simulink model "unit2"  (R2020a)
settings: Solver=VariableStepAuto  StartTime=0.0  StopTime=10.0  RelTol=1e-3
settings Model: Creator=fsepcke  LastModifiedBy=fsepcke

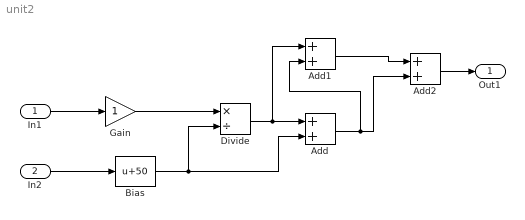
== system unit2 ==
  In1 : Inport
  In2 : Inport  Port=2
  Add : Sum
  Add1 : Sum
  Add2 : Sum
  Bias : Bias  Bias=50
  Divide : Product  Inputs=*/
  Gain : Gain
  Out1 : Outport
  wires:
  In2/1 -> Bias/1
  Bias/1 -> Add/2, Divide/2
  Add/1 -> Add1/2, Add2/2
  Divide/1 -> Add1/1, Add/1
  Add1/1 -> Add2/1
  Add2/1 -> Out1/1
  Gain/1 -> Divide/1
  In1/1 -> Gain/1
